simulink model "three_sign_conventions"  (R2021a)
settings: Solver=VariableStepAuto  StartTime=0.0  StopTime=10.0  RelTol=1e-3
InitFcn:
  | M=100
  | k=1000
  | b=100
settings Model: Creator=byronmason  LastModifiedBy=byronmason

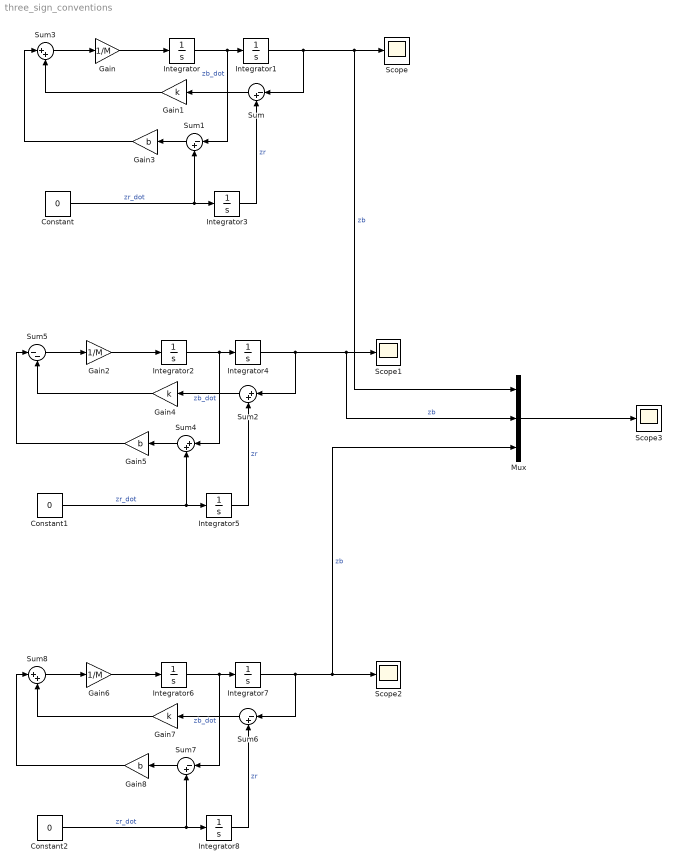
== system three_sign_conventions ==
  Constant : Constant  Value=0
  Constant1 : Constant  Value=0
  Constant2 : Constant  Value=0
  Gain : Gain  Gain=1/M
  Gain1 : Gain  Gain=k
  Gain2 : Gain  Gain=1/M
  Gain3 : Gain  Gain=b
  Gain4 : Gain  Gain=k
  Gain5 : Gain  Gain=b
  Gain6 : Gain  Gain=1/M
  Gain7 : Gain  Gain=k
  Gain8 : Gain  Gain=b
  Integrator{,2..3,5..6,8} (6 alike) : Integrator
  Integrator1 : Integrator  InitialCondition=0.5
  Integrator4 : Integrator  InitialCondition=0.5
  Integrator7 : Integrator  InitialCondition=0.5
  Mux : Mux  Inputs=3
  Scope{,1..3} (4 alike) : Scope
  Sum{,1,6..7} (4 alike) : Sum  Inputs=|-+
  Sum{2..4,8} (4 alike) : Sum  Inputs=|++
  Sum5 : Sum  Inputs=|--
  wires:
  Integrator/1 -> Sum1/1, Integrator1/1  "zb_dot"
  Integrator1/1 -> Mux/1, Scope/1, Sum/1  "zb"
  Gain/1 -> Integrator/1
  Constant/1 -> Integrator3/1, Sum1/2  "zr_dot"
  Sum/1 -> Gain1/1
  Gain1/1 -> Sum3/2
  Integrator3/1 -> Sum/2  "zr"
  Sum1/1 -> Gain3/1
  Gain3/1 -> Sum3/1
  Sum3/1 -> Gain/1
  Sum5/1 -> Gain2/1
  Integrator2/1 -> Sum4/1, Integrator4/1  "zb_dot"
  Integrator4/1 -> Mux/2, Scope1/1, Sum2/1  "zb"
  Constant1/1 -> Integrator5/1, Sum4/2  "zr_dot"
  Integrator5/1 -> Sum2/2  "zr"
  Gain2/1 -> Integrator2/1
  Sum2/1 -> Gain4/1
  Gain4/1 -> Sum5/2
  Sum4/1 -> Gain5/1
  Gain5/1 -> Sum5/1
  Integrator6/1 -> Sum7/1, Integrator7/1  "zb_dot"
  Sum8/1 -> Gain6/1
  Integrator8/1 -> Sum6/2  "zr"
  Constant2/1 -> Integrator8/1, Sum7/2  "zr_dot"
  Integrator7/1 -> Mux/3, Scope2/1, Sum6/1  "zb"
  Sum7/1 -> Gain8/1
  Gain6/1 -> Integrator6/1
  Sum6/1 -> Gain7/1
  Gain7/1 -> Sum8/2
  Gain8/1 -> Sum8/1
  Mux/1 -> Scope3/1
